simulink model "EFPR_HPT_Simulink"  (R2023a)
settings: Solver=VariableStepAuto  StartTime=0.0  StopTime=inf  RelTol=1e-3
undefined symbols (not defined in the file): CR, LF
libraries: instrumentseriallib x2, dspfdesign x1, dspxfrm3 x1
settings Model: Creator=alfon  LastModifiedBy=alfon
settings DebuggingCC: ParameterPrecisionLossMsg=none

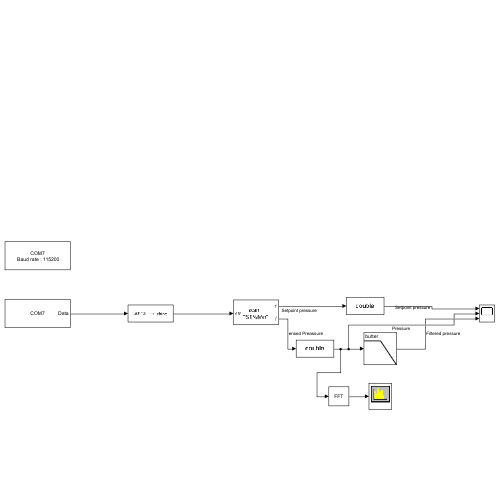
[thumbnail: Simulink's stored preview of the top-level diagram]
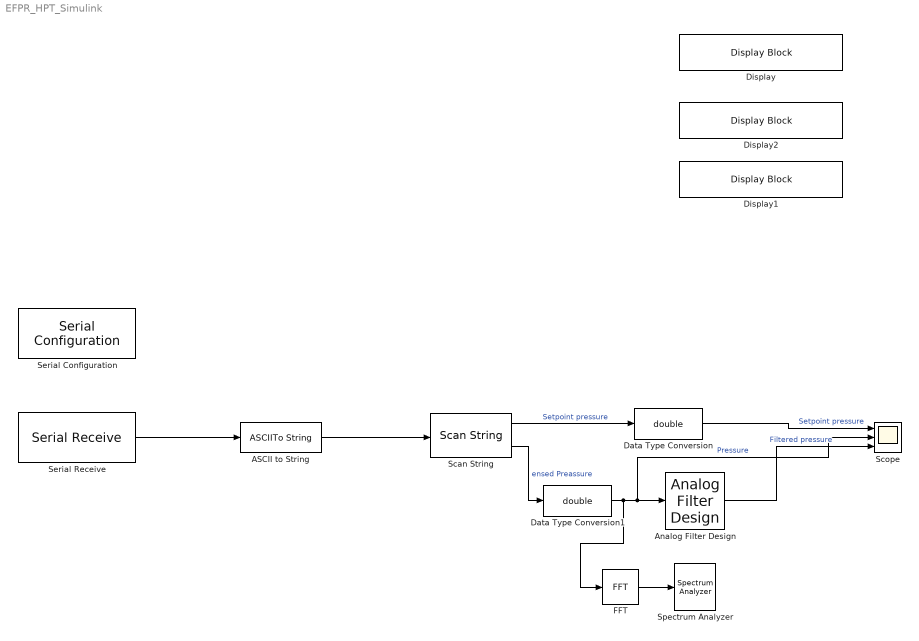
== system EFPR_HPT_Simulink ==
  ASCII to String : ASCIIToString
  Analog Filter Design : dspfdesign/Analog Filter Design  method=Butterworth  filttype=Lowpass  N=8  Wlo=50  Whi=80  Rp=2  Rs=40
  Data Type Conversion : DataTypeConversion  OutDataTypeStr=double  SaturateOnIntegerOverflow=off  RndMeth=Floor
  Data Type Conversion1 : DataTypeConversion  OutDataTypeStr=double  SaturateOnIntegerOverflow=off  RndMeth=Floor
  Display : DisplayBlock  LabelPosition=Hide  Format=Custom  Transparency=1  FormatString=%f
  Display1 : DisplayBlock  LabelPosition=Hide  Format=Custom  Transparency=1  FormatString=%f
  Display2 : DisplayBlock  LabelPosition=Hide  Format=Custom  Transparency=1  FormatString=%f
  FFT : dspxfrm3/FFT  FFTImplementation=Auto  CompMethod=Table lookup  TableOpt=NEW  TableOptActive=Speed  BitRevOrder=off  Normalize=off  InheritFFTLength=on  FFTLength=64  WrapInput=on  roundingMode=Floor  overflowMode=off  firstCoeffDataTypeStr=Inherit: Same word length as input  firstCoeffLastDataTypeStr=Inherit: Same word length as input  outputMin=[]  outputMax=[]
  Scan String : ScanString  Format="\"%f|%f\\r\\n\""
  Scope : Scope  NumInputPorts=3
  Serial Configuration : instrumentseriallib/Serial Configuration  Priority=-200000  PortSel=COM7  Port=COM7  ComPort=COM7  BaudRate=115200  DataBits=8  Parity=none  StopBits=1  ByteOrder=little-endian  FlowControl=none  Timeout=10  SimulateUsing=Interpreted execution  BlockInModel=on  aMode=1
  Serial Receive : instrumentseriallib/Serial Receive  Priority=1  PortSel=COM7  Port=COM7  ComPort=COM7  DataType=uint8  SaveDataType=uint8  ToggleHeader=off  Header=[]  ToggleTerminator=on  Terminator=CR/LF ('\r\n')  CustomTerminator=[]  InputFormat=Column major  ToggleDataSize=on  DataSize=[1 9]  EnableBlockingMode=on  ActionDataUnavailable=Output last received value  ActionWhenDataUnavailable=Output last received value  CustomValue=0  SampleTime=0.001  SimulateUsing=Interpreted execution  BlockInModel=on  aMode=1
  Spectrum Analyzer : SpectrumAnalyzer  WindowPosition=[1.000000,49.000000,2560.000000,1529.000000,]  ScopeFrameLocation=window  YLimits=[-48.70535289,41.27585518]  ColorLimits=[-80 20]
  wires:
  Serial Receive/1 -> ASCII to String/1
  ASCII to String/1 -> Scan String/1
  Scan String/1 -> Data Type Conversion/1  "Setpoint pressure"
  Data Type Conversion/1 -> Scope/1  "Setpoint pressure"
  Data Type Conversion1/1 -> FFT/1, Scope/2, Analog Filter Design/1  "Pressure"
  Scan String/2 -> Data Type Conversion1/1  "ensed Preassure"
  Analog Filter Design/1 -> Scope/3  "Filtered pressure"
  FFT/1 -> Spectrum Analyzer/1
